simulink model "uav"  (R2022b)
settings: Solver=VariableStepAuto  StartTime=0.0  StopTime=10.0  RelTol=1e-3
values from neighbouring files (symbols this model uses):
  Ixx = 1    [variables.m]
  Iyy = 1    [variables.m]
  Izz = 1    [variables.m]
undefined symbols (not defined in the file or in its folder): Ax, Ay, Az, b, d, g, I, Jr, m
libraries: slpidlib x4
settings Model: Creator=0877245  LastModifiedBy=0877245

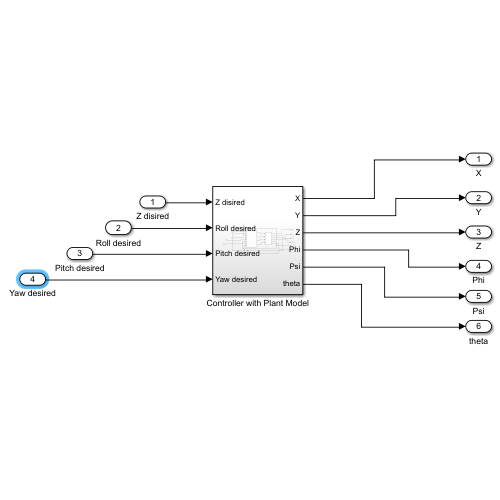
[thumbnail: Simulink's stored preview of the top-level diagram]
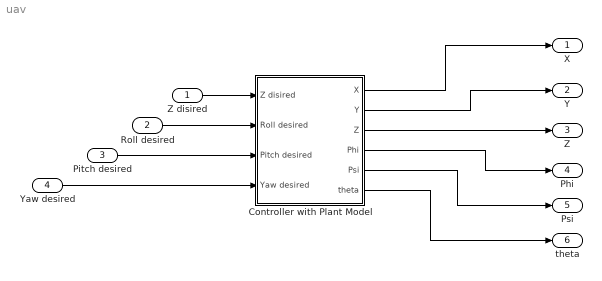
== system uav ==
  Z disired : Inport
  Roll desired : Inport  Port=2
  Pitch desired : Inport  Port=3
  Yaw desired : Inport  Port=4
  "Controller with Plant Model " : Subsystem
  X : Outport
  Y : Outport  Port=2
  Z : Outport  Port=3
  Phi : Outport  Port=4
  Psi : Outport  Port=5
  theta : Outport  Port=6
  wires:
  Z disired/1 -> "Controller with Plant Model "/1(Z disired)
  Roll desired/1 -> "Controller with Plant Model "/2(Roll desired)
  Pitch desired/1 -> "Controller with Plant Model "/3(Pitch desired)
  Yaw desired/1 -> "Controller with Plant Model "/4(Yaw desired)
  "Controller with Plant Model "/1(X) -> X/1
  "Controller with Plant Model "/2(Y) -> Y/1
  "Controller with Plant Model "/3(Z) -> Z/1
  "Controller with Plant Model "/4(Phi) -> Phi/1
  "Controller with Plant Model "/5(Psi) -> Psi/1
  "Controller with Plant Model "/6(theta) -> theta/1

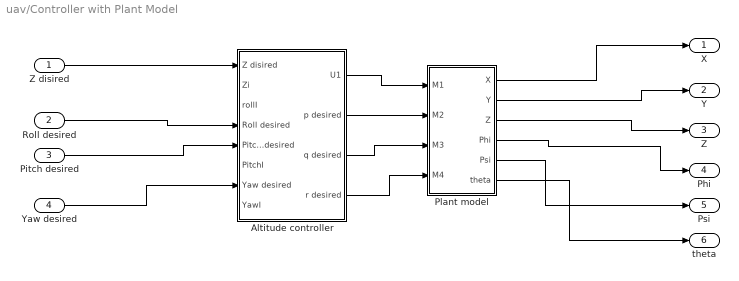
== system uav/Controller with Plant Model  ==
  Z disired : Inport
  Roll desired : Inport  Port=2
  Pitch desired : Inport  Port=3
  Yaw desired : Inport  Port=4
  Altitude controller : Subsystem
  Plant model : Subsystem
  X : Outport
  Y : Outport  Port=2
  Z : Outport  Port=3
  Phi : Outport  Port=4
  Psi : Outport  Port=5
  theta : Outport  Port=6
  wires:
  Plant model/4(Phi) -> Phi/1
  Altitude controller/4(r desired) -> Plant model/4(M4)
  Z disired/1 -> Altitude controller/1(Z disired)
  Altitude controller/2(p desired) -> Plant model/2(M2)
  Plant model/1(X) -> X/1
  Roll desired/1 -> Altitude controller/4(Roll desired)
  Altitude controller/3(q desired) -> Plant model/3(M3)
  Plant model/6(theta) -> theta/1
  Plant model/3(Z) -> Z/1
  Plant model/2(Y) -> Y/1
  Altitude controller/1(U1) -> Plant model/1(M1)
  Plant model/5(Psi) -> Psi/1
  Yaw desired/1 -> Altitude controller/7(Yaw desired)
  Pitch desired/1 -> Altitude controller/5(Pitch desired)

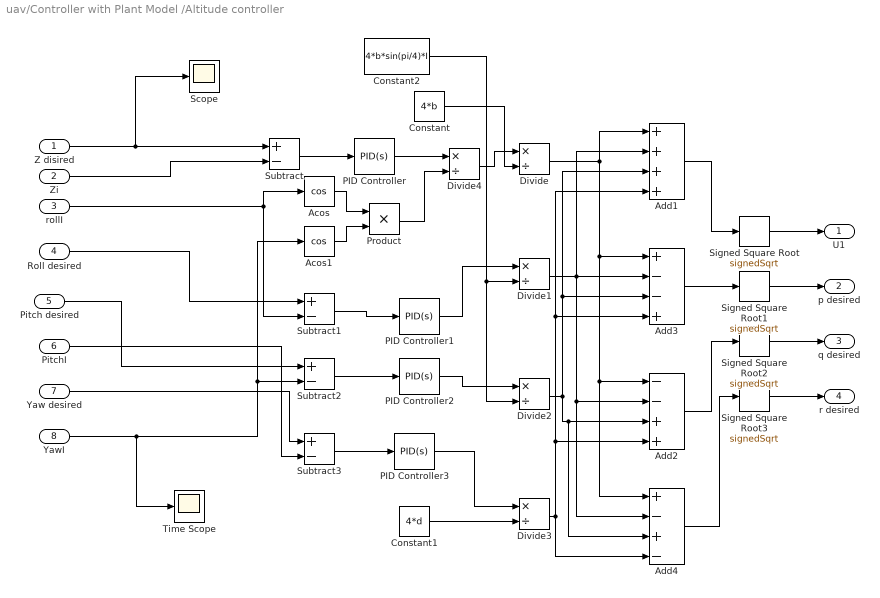
== system uav/Controller with Plant Model /Altitude controller ==
  Z disired : Inport
  Zi : Inport  Port=2
  rollI : Inport  Port=3
  Roll desired : Inport  Port=4
  Pitch desired : Inport  Port=5
  PitchI : Inport  Port=6
  Yaw desired : Inport  Port=7
  YawI : Inport  Port=8
  Acos : Trigonometry  Operator=cos
  Acos1 : Trigonometry  Operator=cos
  Add1 : Sum  Inputs=++++
  Add2 : Sum  Inputs=--++
  Add3 : Sum  Inputs=+--+
  Add4 : Sum  Inputs=+-+-
  Constant : Constant  Value=4*b
  Constant1 : Constant  Value=4*d
  Constant2 : Constant  Value=4*b*sin(pi/4)*I
  Divide{,1..4} (5 alike) : Product  Inputs=*/
  PID Controller{,1..3} (4 alike) : slpidlib/PID Controller  Controller=PID  Form=Parallel  TimeDomain=Continuous-time  UseExternalTs=off  SampleTime=-1  IntegratorMethod=Forward Euler  FilterMethod=Forward Euler  ControllerParametersSource=internal  P=1  I=1  UseKiTs=off  D=0  N=100  UseFilter=on  TunerSelectOption=Transfer Function Based (PID Tuner App)  InitialConditionSource=internal  InitialConditionForIntegrator=0  InitialConditionForFilter=0  DifferentiatorICPrevScaledInput=0  ExternalReset=none  TrackingMode=off  Kt=1  LimitOutput=off  SatLimitsSource=internal  UpperSaturationLimit=inf  LowerSaturationLimit=-inf  LinearizeAsGain=on  AntiWindupMode=none  Kb=1  LimitIntegrator=off  UpperIntegratorSaturationLimit=inf  LowerIntegratorSaturationLimit=-inf  POutMin=[]  POutMax=[]  IOutMin=[]  IOutMax=[]  DOutMin=[]  DOutMax=[]  NOutMin=[]  NOutMax=[]  SumOutMin=[]  SumOutMax=[]  SaturationOutMin=[]  SaturationOutMax=[]  PParamMin=[]  PParamMax=[]  IParamMin=[]  IParamMax=[]  DParamMin=[]  DParamMax=[]  NParamMin=[]  NParamMax=[]  KbParamMin=[]  KbParamMax=[]  KtParamMin=[]  KtParamMax=[]  KbOutMin=[]  KbOutMax=[]  KtOutMin=[]  KtOutMax=[]  IntegratorOutMin=[]  IntegratorOutMax=[]  FilterOutMin=[]  FilterOutMax=[]  SumI1OutMin=[]  SumI1OutMax=[]  SumI2OutMin=[]  SumI2OutMax=[]  SumI3OutMin=[]  SumI3OutMax=[]  SumI4OutMin=[]  SumI4OutMax=[]  SumDOutMin=[]  SumDOutMax=[]  DifferentiatorOutMin=[]  DifferentiatorOutMax=[]  FilterDiffOutCoefMin=[]  FilterDiffOutCoefMax=[]  ReciprocalOutMin=[]  ReciprocalOutMax=[]  SumDenOutMin=[]  SumDenOutMax=[]  SumNumOutMin=[]  SumNumOutMax=[]  DivideOutMin=[]  DivideOutMax=[]  UdiffTsProdOutMin=[]  UdiffTsProdOutMax=[]  NTsProdOutMin=[]  NTsProdOutMax=[]  UintegralTsProdOutMin=[]  UintegralTsProdOutMax=[]  UngainTsProdOutMin=[]  UngainTsProdOutMax=[]  ClampingZeroOutDataTypeStr=Inherit: Inherit via back propagation  ClampingZeroOutMin=[]  ClampingZeroOutMax=[]  FilterDenConstantOutDataTypeStr=Inherit: Inherit via back propagation  FilterDenConstantOutMin=[]  FilterDenConstantOutMax=[]  PCopyOutDataTypeStr=Inherit: Inherit via back propagation  PCopyOutMin=[]  PCopyOutMax=[]  NCopyOutDataTypeStr=Inherit: Inherit via back propagation  NCopyOutMin=[]  NCopyOutMax=[]  IntegratorContinuousStateAttributes=''  IntegratorStateMustResolveToSignalObject=off  IntegratorRTWStateStorageClass=Auto  FilterContinuousStateAttributes=''  FilterStateMustResolveToSignalObject=off  FilterRTWStateStorageClass=Auto  ParallelPVariant=InternalParameters  IdealPVariant=Disabled  IVariant=InternalParameters  DVariant=InternalParameters  IntegratorVariant=Continuous  SatVariant=Disabled  AWVariant=Passthrough  PCopyVariant=Disabled  TRVariant=Disabled  FdbkBlocksVariant=Forward  IdealPFdbkVariant=Disabled  SatFdbkVariant=Disabled  DerivativeFilterVariant=ContFilter  NVariant=InternalParameters  NCopyVariant=Disabled  FilterICVariant=InternalICsFilter  IntegratorICVariant=InternalICs  ExternalResetVariant=Disabled  TRSumVariant=Passthrough  SumFdbkVariant=Disabled  SumVariant=Sum_PID  TsampFilterVariant=InternalTs  TsampNgainVariant=Passthrough  TsampIntegralVariant=Passthrough  ExternalSaturationOutDataTypeStr=Inherit: Same as second input
  Product : Product
  Scope : Scope
  Signed Square Root{,1..3} (4 alike) : Sqrt  Operator=signedSqrt
  Subtract{,1..3} (4 alike) : Sum  Inputs=+-
  Time Scope : Scope
  U1 : Outport
  p desired : Outport  Port=2
  q desired : Outport  Port=3
  r desired : Outport  Port=4
  wires:
  Divide1/1 -> Add4/2, Add2/2, Add3/2, Add1/2
  PID Controller3/1 -> Divide3/1
  Subtract1/1 -> PID Controller1/1
  Add1/1 -> Signed Square Root/1
  Constant2/1 -> Divide2/2, Divide1/2
  Acos/1 -> Product/1
  Signed Square Root2/1 -> q desired/1
  Divide2/1 -> Add3/3, Add1/3, Add4/3, Add2/3
  Signed Square Root1/1 -> p desired/1
  Product/1 -> Divide4/2
  Add3/1 -> Signed Square Root1/1
  Roll desired/1 -> Subtract1/1
  Divide3/1 -> Add2/4, Add3/4, Add1/4, Add4/4
  PitchI/1 -> Subtract3/2
  Add2/1 -> Signed Square Root2/1
  Z disired/1 -> Scope/1, Subtract/1
  Signed Square Root/1 -> U1/1
  Zi/1 -> Subtract/2
  Subtract2/1 -> PID Controller2/1
  Constant1/1 -> Divide3/2
  Subtract3/1 -> PID Controller3/1
  Divide/1 -> Add1/1, Add4/1, Add2/1, Add3/1
  PID Controller/1 -> Divide4/1
  Add4/1 -> Signed Square Root3/1
  Acos1/1 -> Product/2
  PID Controller2/1 -> Divide2/1
  rollI/1 -> Subtract1/2, Acos/1
  Subtract/1 -> PID Controller/1
  Divide4/1 -> Divide/1
  Constant/1 -> Divide/2
  Pitch desired/1 -> Subtract2/1
  PID Controller1/1 -> Divide1/1
  Yaw desired/1 -> Subtract3/1
  YawI/1 -> Time Scope/1, Subtract2/2, Acos1/1
  Signed Square Root3/1 -> r desired/1

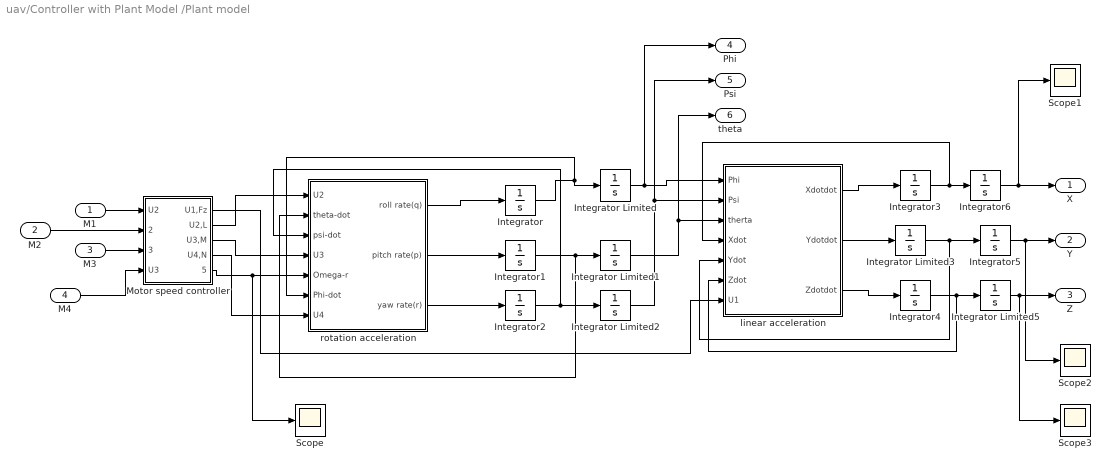
== system uav/Controller with Plant Model /Plant model ==
  M1 : Inport
  M2 : Inport  Port=2
  M3 : Inport  Port=3
  M4 : Inport  Port=4
  Integrator{,1..6} (7 alike) : Integrator
  Integrator Limited{,1..3,5} (5 alike) : Integrator  LimitOutput=on  UpperSaturationLimit=1  LowerSaturationLimit=0
  Motor speed controller : Subsystem
  Scope{,1..3} (4 alike) : Scope
  linear acceleration : Subsystem
  rotation acceleration : Subsystem
  X : Outport
  Y : Outport  Port=2
  Z : Outport  Port=3
  Phi : Outport  Port=4
  Psi : Outport  Port=5
  theta : Outport  Port=6
  wires:
  Integrator5/1 -> Y/1, Scope2/1
  Integrator6/1 -> X/1, Scope1/1
  Integrator2/1 -> rotation acceleration/3(psi-dot), Integrator Limited2/1
  Motor speed controller/5(Omega) -> Scope/1, rotation acceleration/5(Omega-r)
  Integrator Limited3/1 -> linear acceleration/5(Ydot), Integrator5/1
  linear acceleration/3(Zdotdot) -> Integrator4/1
  Motor speed controller/3(U3,M) -> rotation acceleration/4(U3)
  Integrator3/1 -> linear acceleration/4(Xdot), Integrator6/1
  M1/1 -> Motor speed controller/1(U2)
  Motor speed controller/4(U4,N) -> rotation acceleration/7(U4)
  Integrator Limited5/1 -> Z/1, Scope3/1
  Integrator/1 -> rotation acceleration/6(Phi-dot), Integrator Limited/1
  linear acceleration/2(Ydotdot) -> Integrator Limited3/1
  Integrator Limited/1 -> Phi/1, linear acceleration/1(Phi)
  Integrator4/1 -> linear acceleration/6(Zdot), Integrator Limited5/1
  M4/1 -> Motor speed controller/4(U3)
  Integrator Limited2/1 -> Psi/1, linear acceleration/2(Psi)
  M2/1 -> Motor speed controller/2(theta-dot)
  Motor speed controller/1(U1,Fz) -> linear acceleration/7(U1)
  Motor speed controller/2(U2,L) -> rotation acceleration/1(U2)
  Integrator Limited1/1 -> theta/1, linear acceleration/3(therta)
  Integrator1/1 -> rotation acceleration/2(theta-dot), Integrator Limited1/1
  rotation acceleration/3(yaw rate(r)) -> Integrator2/1
  rotation acceleration/1(roll rate(q)) -> Integrator/1
  rotation acceleration/2(pitch rate(p)) -> Integrator1/1
  linear acceleration/1(Xdotdot) -> Integrator3/1
  M3/1 -> Motor speed controller/3(psi-dot)

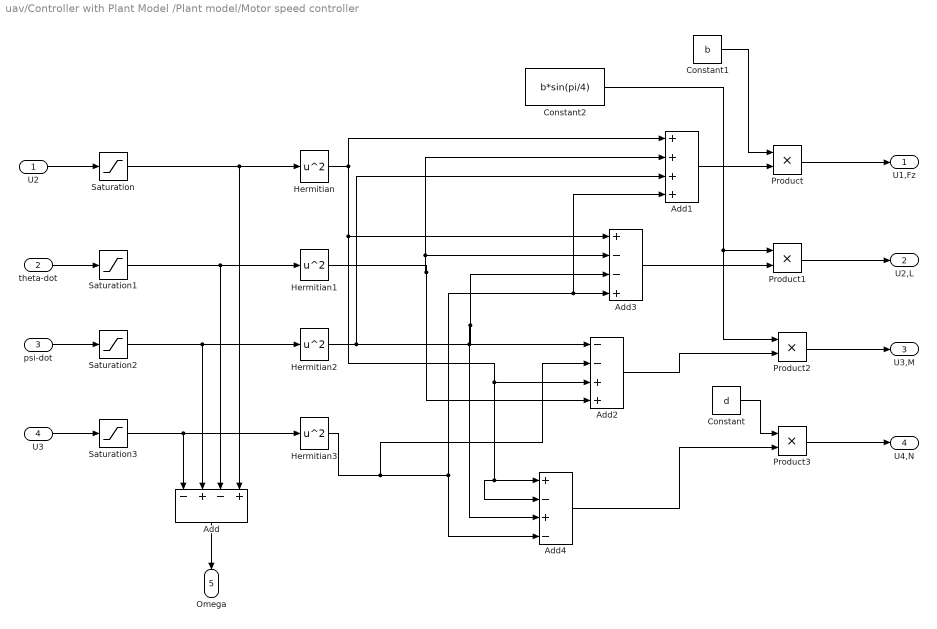
== system uav/Controller with Plant Model /Plant model/Motor speed controller ==
  U2 : Inport
  theta-dot : Inport  Port=2
  psi-dot : Inport  Port=3
  U3 : Inport  Port=4
  Add : Sum  Inputs=-+-+
  Add1 : Sum  Inputs=++++
  Add2 : Sum  Inputs=--++
  Add3 : Sum  Inputs=+--+
  Add4 : Sum  Inputs=+-+-
  Constant : Constant  Value=d
  Constant1 : Constant  Value=b
  Constant2 : Constant  Value=b*sin(pi/4)
  Hermitian{,1..3} (4 alike) : Math  Operator=square
  Product{,1..3} (4 alike) : Product
  Saturation{,1..3} (4 alike) : Saturate
  U1,Fz : Outport
  U2,L : Outport  Port=2
  U3,M : Outport  Port=3
  U4,N : Outport  Port=4
  Omega : Outport  Port=5
  wires:
  theta-dot/1 -> Saturation1/1
  U2/1 -> Saturation/1
  psi-dot/1 -> Saturation2/1
  U3/1 -> Saturation3/1
  Saturation3/1 -> Hermitian3/1, Add/1
  Saturation2/1 -> Hermitian2/1, Add/2
  Saturation1/1 -> Hermitian1/1, Add/3
  Saturation/1 -> Add/4, Hermitian/1
  Product/1 -> U1,Fz/1
  Product1/1 -> U2,L/1
  Product2/1 -> U3,M/1
  Product3/1 -> U4,N/1
  Hermitian/1 -> Add4/2, Add4/1, Add2/3, Add3/1, Add1/1
  Add1/1 -> Product/2
  Add3/1 -> Product1/2
  Add2/1 -> Product2/2
  Add4/1 -> Product3/2
  Hermitian1/1 -> Add1/2, Add3/2, Add2/4
  Hermitian2/1 -> Add1/3, Add4/3, Add3/3, Add2/1
  Hermitian3/1 -> Add2/2, Add1/4, Add3/4, Add4/4
  Constant/1 -> Product3/1
  Constant1/1 -> Product/1
  Constant2/1 -> Product2/1, Product1/1
  Add/1 -> Omega/1

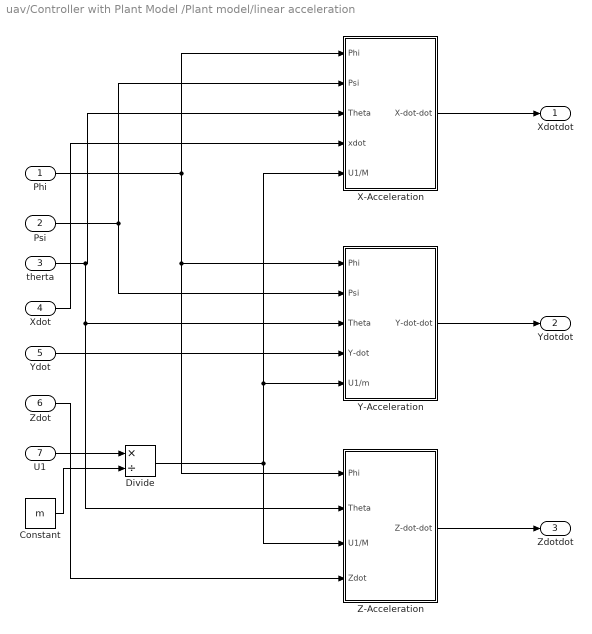
== system uav/Controller with Plant Model /Plant model/linear acceleration ==
  Phi : Inport
  Psi : Inport  Port=2
  therta : Inport  Port=3
  Xdot : Inport  Port=4
  Ydot : Inport  Port=5
  Zdot : Inport  Port=6
  U1 : Inport  Port=7
  " X-Acceleration " : Subsystem
  " Y-Acceleration " : Subsystem
  Constant : Constant  Value=m
  Divide : Product  Inputs=*/
  "Z-Acceleration " : Subsystem
  Xdotdot : Outport
  Ydotdot : Outport  Port=2
  Zdotdot : Outport  Port=3
  wires:
  therta/1 -> "Z-Acceleration "/2(Theta), " Y-Acceleration "/3(Theta), " X-Acceleration "/3(Theta)
  " X-Acceleration "/1(X-dot-dot) -> Xdotdot/1
  " Y-Acceleration "/1(Y-dot-dot) -> Ydotdot/1
  "Z-Acceleration "/1(Z-dot-dot) -> Zdotdot/1
  Phi/1 -> "Z-Acceleration "/1(Phi), " Y-Acceleration "/1(Phi), " X-Acceleration "/1(Phi)
  Psi/1 -> " X-Acceleration "/2(Psi), " Y-Acceleration "/2(Psi)
  Xdot/1 -> " X-Acceleration "/4(xdot)
  Zdot/1 -> "Z-Acceleration "/4(Zdot)
  Ydot/1 -> " Y-Acceleration "/4(Y-dot)
  Divide/1 -> " Y-Acceleration "/5(U1/m), " X-Acceleration "/5(U1/M), "Z-Acceleration "/3(U1/M)
  U1/1 -> Divide/1
  Constant/1 -> Divide/2

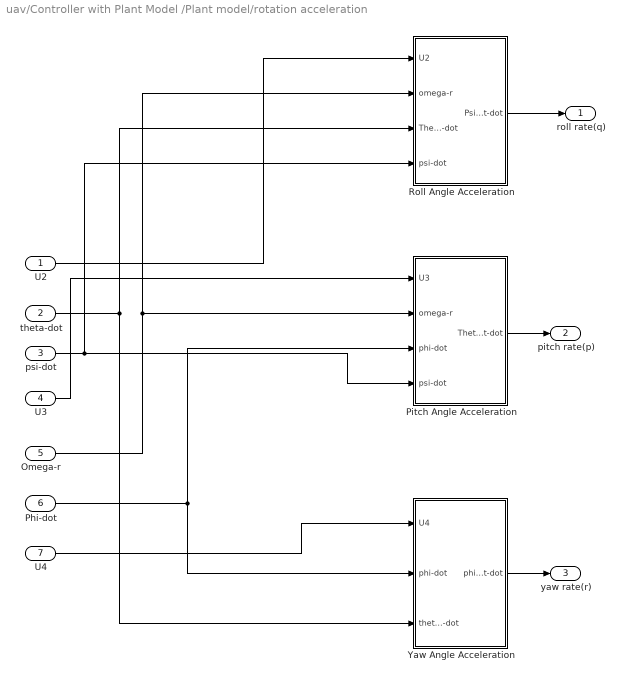
== system uav/Controller with Plant Model /Plant model/rotation acceleration ==
  U2 : Inport
  theta-dot : Inport  Port=2
  psi-dot : Inport  Port=3
  U3 : Inport  Port=4
  Omega-r : Inport  Port=5
  Phi-dot : Inport  Port=6
  U4 : Inport  Port=7
  "  Pitch Angle Acceleration" : Subsystem
  "  Yaw Angle Acceleration" : Subsystem
  " Roll Angle Acceleration" : Subsystem
  roll rate(q) : Outport
  pitch rate(p) : Outport  Port=2
  yaw rate(r) : Outport  Port=3
  wires:
  " Roll Angle Acceleration"/1(Psi-dot-dot) -> roll rate(q)/1
  theta-dot/1 -> " Roll Angle Acceleration"/3(Theta-dot), "  Yaw Angle Acceleration"/3(theta-dot)
  Omega-r/1 -> "  Pitch Angle Acceleration"/2(omega-r), " Roll Angle Acceleration"/2(omega-r)
  "  Yaw Angle Acceleration"/1(phi-dot-dot) -> yaw rate(r)/1
  Phi-dot/1 -> "  Yaw Angle Acceleration"/2(phi-dot), "  Pitch Angle Acceleration"/3(phi-dot)
  U3/1 -> "  Pitch Angle Acceleration"/1(U3)
  psi-dot/1 -> " Roll Angle Acceleration"/4(psi-dot), "  Pitch Angle Acceleration"/4(psi-dot)
  U2/1 -> " Roll Angle Acceleration"/1(U2)
  U4/1 -> "  Yaw Angle Acceleration"/1(U4)
  "  Pitch Angle Acceleration"/1(Thetai-dot-dot) -> pitch rate(p)/1

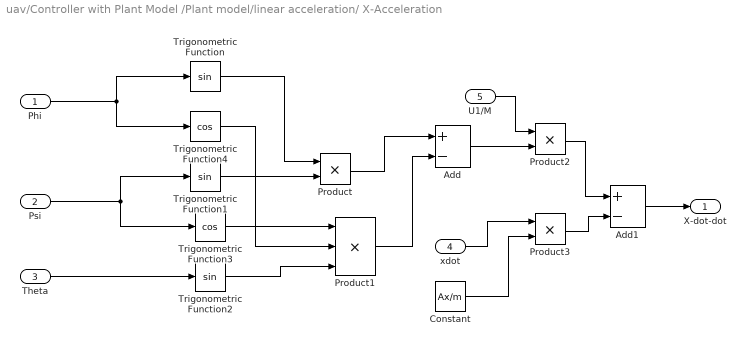
== system uav/Controller with Plant Model /Plant model/linear acceleration/ X-Acceleration  ==
  Phi : Inport
  Psi : Inport  Port=2
  Theta : Inport  Port=3
  xdot : Inport  Port=4
  U1/M : Inport  Port=5
  Add : Sum  Inputs=+-
  Add1 : Sum  Inputs=+-
  Constant : Constant  Value=Ax/m
  Product : Product
  Product1 : Product  Inputs=3
  Product2 : Product
  Product3 : Product
  Trigonometric Function : Trigonometry
  Trigonometric Function1 : Trigonometry
  Trigonometric Function2 : Trigonometry
  Trigonometric Function3 : Trigonometry  Operator=cos
  Trigonometric Function4 : Trigonometry  Operator=cos
  X-dot-dot : Outport
  wires:
  Product/1 -> Add/1
  Product1/1 -> Add/2
  Trigonometric Function/1 -> Product/1
  Trigonometric Function4/1 -> Product1/2
  Trigonometric Function1/1 -> Product/2
  Trigonometric Function3/1 -> Product1/1
  Trigonometric Function2/1 -> Product1/3
  Product2/1 -> Add1/1
  Product3/1 -> Add1/2
  Add1/1 -> X-dot-dot/1
  Constant/1 -> Product3/2
  xdot/1 -> Product3/1
  Phi/1 -> Trigonometric Function/1, Trigonometric Function4/1
  Psi/1 -> Trigonometric Function1/1, Trigonometric Function3/1
  Theta/1 -> Trigonometric Function2/1
  U1/M/1 -> Product2/1
  Add/1 -> Product2/2

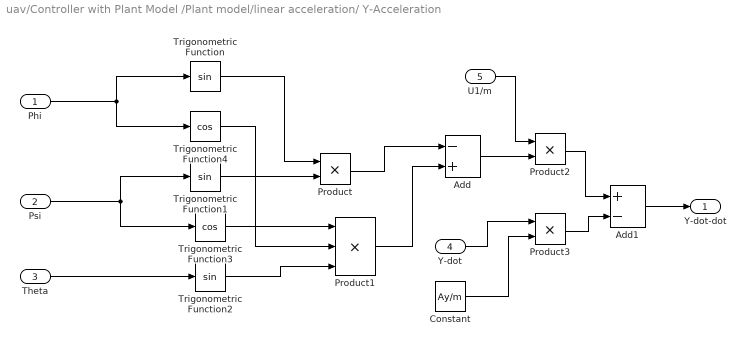
== system uav/Controller with Plant Model /Plant model/linear acceleration/ Y-Acceleration  ==
  Phi : Inport
  Psi : Inport  Port=2
  Theta : Inport  Port=3
  Y-dot : Inport  Port=4
  U1/m : Inport  Port=5
  Add : Sum  Inputs=-+
  Add1 : Sum  Inputs=+-
  Constant : Constant  Value=Ay/m
  Product : Product
  Product1 : Product  Inputs=3
  Product2 : Product
  Product3 : Product
  Trigonometric Function : Trigonometry
  Trigonometric Function1 : Trigonometry
  Trigonometric Function2 : Trigonometry
  Trigonometric Function3 : Trigonometry  Operator=cos
  Trigonometric Function4 : Trigonometry  Operator=cos
  Y-dot-dot : Outport
  wires:
  Product/1 -> Add/1
  Product1/1 -> Add/2
  Trigonometric Function/1 -> Product/1
  Trigonometric Function4/1 -> Product1/2
  Trigonometric Function1/1 -> Product/2
  Trigonometric Function3/1 -> Product1/1
  Trigonometric Function2/1 -> Product1/3
  Product2/1 -> Add1/1
  Product3/1 -> Add1/2
  Add1/1 -> Y-dot-dot/1
  Constant/1 -> Product3/2
  Y-dot/1 -> Product3/1
  Phi/1 -> Trigonometric Function/1, Trigonometric Function4/1
  Psi/1 -> Trigonometric Function1/1, Trigonometric Function3/1
  Theta/1 -> Trigonometric Function2/1
  U1/m/1 -> Product2/1
  Add/1 -> Product2/2

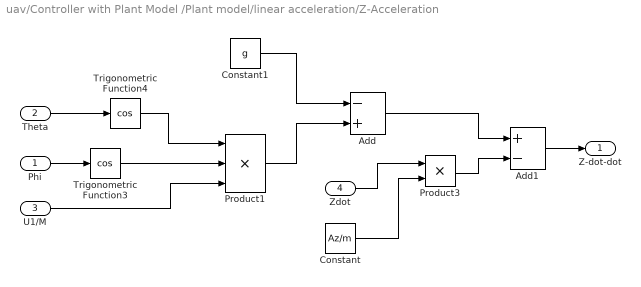
== system uav/Controller with Plant Model /Plant model/linear acceleration/Z-Acceleration  ==
  Phi : Inport
  Theta : Inport  Port=2
  U1/M : Inport  Port=3
  Zdot : Inport  Port=4
  Add : Sum  Inputs=-+
  Add1 : Sum  Inputs=+-
  Constant : Constant  Value=Az/m
  Constant1 : Constant  Value=g
  Product1 : Product  Inputs=3
  Product3 : Product
  Trigonometric Function3 : Trigonometry  Operator=cos
  Trigonometric Function4 : Trigonometry  Operator=cos
  Z-dot-dot : Outport
  wires:
  Product1/1 -> Add/2
  Product3/1 -> Add1/2
  Add1/1 -> Z-dot-dot/1
  Constant/1 -> Product3/2
  Zdot/1 -> Product3/1
  Theta/1 -> Trigonometric Function4/1
  Phi/1 -> Trigonometric Function3/1
  Constant1/1 -> Add/1
  Add/1 -> Add1/1
  U1/M/1 -> Product1/3
  Trigonometric Function4/1 -> Product1/1
  Trigonometric Function3/1 -> Product1/2

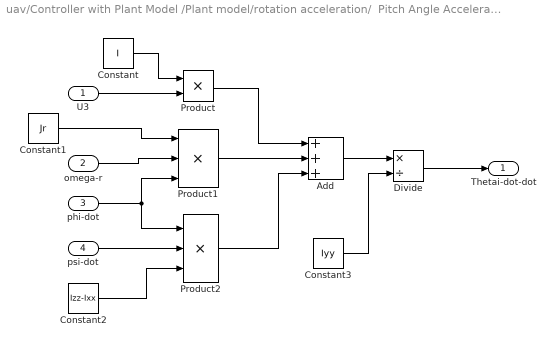
== system uav/Controller with Plant Model /Plant model/rotation acceleration/  Pitch Angle Acceleration ==
  U3 : Inport
  omega-r : Inport  Port=2
  phi-dot : Inport  Port=3
  psi-dot : Inport  Port=4
  Add : Sum  Inputs=+++
  Constant : Constant  Value=I
  Constant1 : Constant  Value=Jr
  Constant2 : Constant  Value=Izz-Ixx
  Constant3 : Constant  Value=Iyy
  Divide : Product  Inputs=*/
  Product : Product
  Product1 : Product  Inputs=3
  Product2 : Product  Inputs=3
  Thetai-dot-dot : Outport
  wires:
  psi-dot/1 -> Product2/2
  Product2/1 -> Add/3
  Constant3/1 -> Divide/2
  Divide/1 -> Thetai-dot-dot/1
  Product/1 -> Add/1
  phi-dot/1 -> Product1/3, Product2/1
  U3/1 -> Product/2
  omega-r/1 -> Product1/2
  Constant2/1 -> Product2/3
  Product1/1 -> Add/2
  Constant1/1 -> Product1/1
  Constant/1 -> Product/1
  Add/1 -> Divide/1

== system uav/Controller with Plant Model /Plant model/rotation acceleration/  Yaw Angle Acceleration ==
  U4 : Inport
  phi-dot : Inport  Port=2
  theta-dot : Inport  Port=3
  Add : Sum
  Constant2 : Constant  Value=Ixx-Izz
  Constant3 : Constant  Value=Izz
  Divide : Product  Inputs=*/
  Product1 : Product  Inputs=3
  phi-dot-dot : Outport
  wires:
  Constant3/1 -> Divide/2
  Divide/1 -> phi-dot-dot/1
  Product1/1 -> Add/2
  Add/1 -> Divide/1
  U4/1 -> Add/1
  Constant2/1 -> Product1/3
  phi-dot/1 -> Product1/1
  theta-dot/1 -> Product1/2

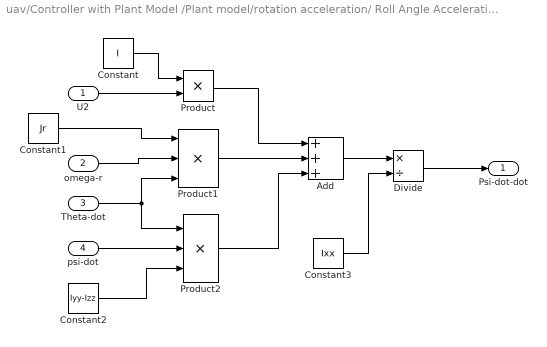
== system uav/Controller with Plant Model /Plant model/rotation acceleration/ Roll Angle Acceleration ==
  U2 : Inport
  omega-r : Inport  Port=2
  Theta-dot : Inport  Port=3
  psi-dot : Inport  Port=4
  Add : Sum  Inputs=+++
  Constant : Constant  Value=I
  Constant1 : Constant  Value=Jr
  Constant2 : Constant  Value=Iyy-Izz
  Constant3 : Constant  Value=Ixx
  Divide : Product  Inputs=*/
  Product : Product
  Product1 : Product  Inputs=3
  Product2 : Product  Inputs=3
  Psi-dot-dot : Outport
  wires:
  psi-dot/1 -> Product2/2
  Product2/1 -> Add/3
  Constant3/1 -> Divide/2
  Divide/1 -> Psi-dot-dot/1
  Product/1 -> Add/1
  Theta-dot/1 -> Product1/3, Product2/1
  U2/1 -> Product/2
  omega-r/1 -> Product1/2
  Constant2/1 -> Product2/3
  Product1/1 -> Add/2
  Constant1/1 -> Product1/1
  Constant/1 -> Product/1
  Add/1 -> Divide/1
